simulink subsystem "Battery_Model"  (R2021b)
settings: Solver=VariableStepAuto  StartTime=0.0  StopTime=10.0  RelTol=1e-3
undefined symbols (not defined in the file): Battery, Np_Module
libraries: fl_lib x580, nesl_utility x386, ee_lib x96, simulink x96
(part 4 of 6)

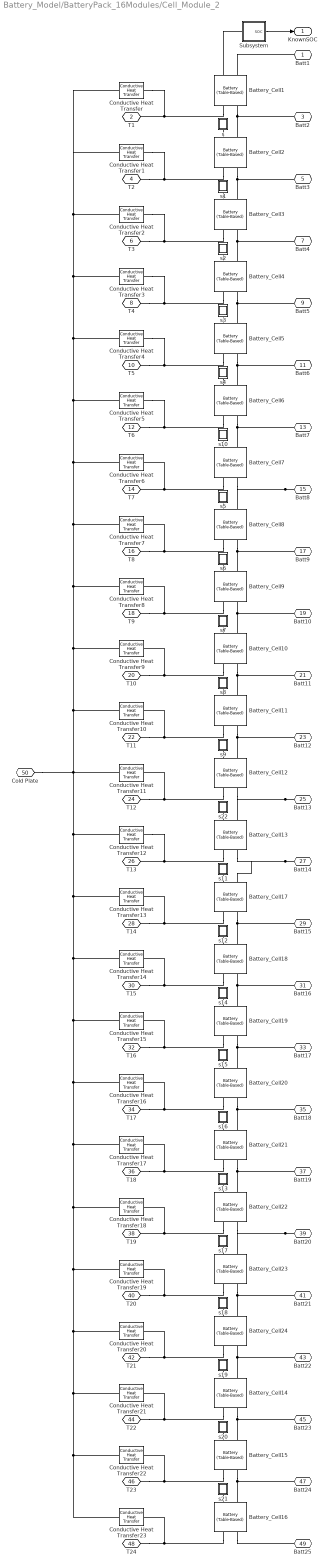
== system Battery_Model/BatteryPack_16Modules/Cell_Module_2 ==
  Battery_Cell{1..24} (24 alike) : ee_lib/Sources/Battery (Table-Based)  Tag={'toolbox/physmod/elec/library/m/ee_lib_parts';'Sources/Battery__Table_Based_/Panasonic/NCR18650BD.xml'}  SOC_vec=Battery.SOC_LUT  T_dependence=ee.enum.temperature_dependence.yes  prm_dir=ee.enum.battery.prm_dir.noCurrentDirectionality  T_vec=Battery.Temperature_LUT degC  V0_mat=Battery.Em_LUT V  V0_vec=[3.01162183959268 3.08575650269622 3.14177499163339 3.18631823552003 3.22334954767724 3.25390136234099 3.27878869705109 3.30070350874259 3.32118523630503 3.33873222862982 3.35681278765286 3.3727103181478 3.38793252475269 3.40246133852855 3.41323877471787 3.42274053961048 3.43230513033606 3.44127066639713 3.45046092538443 3.46050021597496 3.47059444208772 3.47754582201769 3.48403887676592 3.49083263175798 3.49762638675004 3.50414427848956 3.51006189737342 3.51650779121088 3.52300031605604 3.5294928409012 3.53574150484027 3.54126505716735 3.54599126111241 3.55084210438451 3.55569196094666 3.56052372392349 3.56532059653064 3.56979945432131 3.57444121267711 3.57904303346503 3.58364485425295 3.58840361874736 3.5931676308725 3.59914045642067 3.60536834334135 3.61166009904557 3.61797346412467 3.62428682920377 3.63060019428287 3.63762035332317 3.64493091713641 3.65193784155324 3.65894476597006 3.66595169038689 3.67346631195551 3.68205597286888 3.69093403907072 3.69981210527255 3.70876940774879 3.71776352136613 3.72686785650522 3.73538877817079 3.74389655120326 3.7524031927436 3.76046489817023 3.76888762106825 3.7779024493972 3.78684332393235 3.7957841984675 3.80453642296868 3.81235798589345 3.82032795054979 3.82829600796219 3.83626406537459 3.84436267545786 3.8525073311682 3.86057855536852 3.86864977956884 3.87672100376915 3.8849361052788 3.89310639828889 3.90173837211625 3.91095173577988 3.92144530461468 3.93240377767841 3.94373568413835 3.95558619350771 3.96743304428185 3.9792002957498 3.99089798499065 4.00334195302942 4.01527114968024 4.0272843604214 4.03909414300309 4.04916289177822 4.05870791988182 4.06775178122738 4.07651000374835 4.08674414955216 4.1040722856973] V  R0_mat=Battery.R0_LUT/Np_Module Ohm  R0_vec=[0.108383589577359 0.104276452250663 0.0975073630060557 0.0937501268832217 0.0893819468578965 0.085464471367626 0.08175755280038 0.0789657156023766 0.0763700410896049 0.0743500050394976 0.0728433546029721 0.0716898267238282 0.0709947524858037 0.0701675330798173 0.0687296636498531 0.0673712307537144 0.066215812656778 0.0650205672726791 0.0638581443118 0.0632667622677965 0.0628323749302964 0.0619127995096651 0.0610362875653991 0.0603620203223802 0.0596877530793609 0.0589554578065767 0.0582121279560432 0.0577538001128373 0.0573051863053595 0.0568565724978818 0.0563566623767877 0.055788965071129 0.0551527157042777 0.0546601636283963 0.0541676729953156 0.0536763090566326 0.0531776059040765 0.0526119236645948 0.0520712300263528 0.0515036752143958 0.0509361204024388 0.0503587926465561 0.0497811381187243 0.0494179007317461 0.0491061102549 0.0488178197046287 0.0485440631684004 0.0482703066321726 0.0479965500959447 0.0478381475470897 0.0477067926990284 0.0473712163371034 0.0470356399751788 0.0467000636132555 0.0464310667647791 0.0463210072143654 0.0462716139198203 0.0462222206252756 0.0462261199933538 0.0462489440940042 0.0463125045945074 0.0462585966454419 0.046201922872132 0.046144488080849 0.0458836890808221 0.0457208666912199 0.0456935258730669 0.0456707901856075 0.0456480544981481 0.0455856361429716 0.0453236882021848 0.0450859495122442 0.0448483295871047 0.0446107096619652 0.0444608967355156 0.0443618965142365 0.0442474499230245 0.0441330033318126 0.0440185567406002 0.0437935866730954 0.0434800673484186 0.0432636629093239 0.0431695542324042 0.0433145404237085 0.043616651255713 0.0439115402259742 0.0443155176840522 0.0447170344474341 0.0451426585495343 0.0455784262459233 0.0461653340876942 0.0463666936277911 0.0465478472510501 0.0466774333752156 0.0460938543815081 0.045231226285297 0.0442160431848739 0.0431407757562075 0.0415552249991693 0.0395514196760085] Ohm  R0_dis_mat=[0.03 0.015 0.002;0.04 0.017 0.008;0.039 0.012 0.006;0.027 0.013 0.021] % Parameter not set Ohm  R0_dis_vec=[0.015 0.017 0.012 0.013] % Parameter not set Ohm  R0_ch_mat=[0.03 0.015 0.002;0.04 0.017 0.008;0.039 0.012 0.006;0.027 0.013 0.021] % Parameter not set Ohm  R0_ch_vec=[0.015 0.017 0.012 0.013] % Parameter not set Ohm  AH_vec=Battery.Capacity_LUT*Np_Module hr*A  AH=3.03732766876938 hr*A  prm_leak=ee.enum.battery.prm_leak.disabled  Rleak_vec=[8000 7000 6000] % Parameter not set Ohm  Rleak=7000 % Parameter not set Ohm  extrapolation_option=ee.enum.extrapolation.nearest  prm_dyn=ee.enum.battery.prm_dyn.rc1  R1_mat=Battery.R1_LUT/Np_Module Ohm  R1_vec=[0.076 0.022 0.007 0.043] % Parameter not set Ohm  tau1_mat=(Battery.R1_LUT/Np_Module).*(Battery.C1_LUT*Np_Module) s  tau1_vec=[148 110 27 22] % Parameter not set s  R2_mat=[0.014 0.382 0.407;0.028 0.006 0.007;0.014 0.007 0.006;0.333 0.956 0.912] % Parameter not set Ohm  R2_vec=[0.382 0.006 0.007 0.956] % Parameter not set Ohm  tau2_mat=[1 44 5644;11 24 506;2 14 330;3310 13419 30216] % Parameter not set s  tau2_vec=[44 24 14 13419] % Parameter not set s  R3_mat=[0.014 0.382 0.407;0.028 0.006 0.007;0.014 0.007 0.006;0.333 0.956 0.912] % Parameter not set Ohm  R3_vec=[0.382 0.006 0.007 0.956] % Parameter not set Ohm  tau3_mat=[1 44 5644;11 24 506;2 14 330;3310 13419 30216] % Parameter not set s  tau3_vec=[44 24 14 13419] % Parameter not set s  R4_mat=[0.014 0.382 0.407;0.028 0.006 0.007;0.014 0.007 0.006;0.333 0.956 0.912] % Parameter not set Ohm  R4_vec=[0.382 0.006 0.007 0.956] % Parameter not set Ohm  tau4_mat=[1 44 5644;11 24 506;2 14 330;3310 13419 30216] % Parameter not set s  tau4_vec=[44 24 14 13419] % Parameter not set s  R5_mat=[0.014 0.382 0.407;0.028 0.006 0.007;0.014 0.007 0.006;0.333 0.956 0.912] % Parameter not set Ohm  R5_vec=[0.382 0.006 0.007 0.956] % Parameter not set Ohm  tau5_mat=[1 44 5644;11 24 506;2 14 330;3310 13419 30216] % Parameter not set s  tau5_vec=[44 24 14 13419] % Parameter not set s  prm_fade=ee.enum.battery.prm_fade.tableN  N0=100 % Parameter not set  dV0=0 % Parameter not set  dR0=0 % Parameter not set  dAH=0 % Parameter not set  dRleak=0 % Parameter not set  dR1=0 % Parameter not set  dR2=0 % Parameter not set  dR3=0 % Parameter not set  dR4=0 % Parameter not set  dR5=0 % Parameter not set  N0vec=Battery.DischargeCycle_LUT  Tfadevec=[298.15 323.15] % Parameter not set K  dV0vec=Battery.deltaEm_LUT  dR0vec=[0;0;0;0;0;0;0;0;0;0;0;0;0;0;0;0;0;0;0;0;0;0;0;0;0;0;0;0;0;0;0;0;0;0;0;0;0;0;0;0;0;0;0;0;0;0;0;0;0;0;0;0;0;0;0;0;0;0;0;0;0;0;0;0;0;0;0;0;0;0;0;0;0;0;0;0;0;0;0;0] % Parameter not set  dAHvec=Battery.deltaCapacity_LUT  dRleakvec=[0 0 0] % Parameter not set  dR1vec=[0;0;0;0;0;0;0;0;0;0;0;0;0;0;0;0;0;0;0;0;0;0;0;0;0;0;0;0;0;0;0;0;0;0;0;0;0;0;0;0;0;0;0;0;0;0;0;0;0;0;0;0;0;0;0;0;0;0;0;0;0;0;0;0;0;0;0;0;0;0;0;0;0;0;0;0;0;0;0;0] % Parameter not set  dR2vec=[0 0 0] % Parameter not set  dR3vec=[0 0 0] % Parameter not set  dR4vec=[0 0 0] % Parameter not set  dR5vec=[0 0 0] % Parameter not set  dV0mat=[0 0;0 0;0 0] % Parameter not set  dR0mat=[0 0;0 0;0 0] % Parameter not set  dAHmat=[0 0;0 0;0 0] % Parameter not set  dRleakmat=[0 0;0 0;0 0] % Parameter not set  dR1mat=[0 0;0 0;0 0] % Parameter not set  dR2mat=[0 0;0 0;0 0] % Parameter not set  dR3mat=[0 0;0 0;0 0] % Parameter not set  dR4mat=[0 0;0 0;0 0] % Parameter not set  dR5mat=[0 0;0 0;0 0] % Parameter not set  prm_age=ee.enum.battery.prm_age.disabled  prm_age_OCV=ee.enum.battery.prm_age_OCV.OCV  OCV_age=0.9  SOC_age=0.6  storage_dt_age_vec=[0] d  storage_T_age_vec=[273] K  OCV_scaling_age=2.2134e6  OCV_offset_age=1.632e6  temp_exp_age=0.515833569 V  t_exp_age=0.75  T_age_vec=[273.15, 298.15, 323.15] K  dt_age_vec=[90, 180, 270, 360] d  dR0_age_vec=[0, 0, 0]  t_meas_dR0_age=100 d  dR0_age_mat=[0, 0, 0; 0, 0, 0; 0, 0, 0; 0, 0, 0]  temperature=BattTempInit degC  i_specify=off  i_priority=None  i=0 A  i_nominal_specify=off  i_nominal_unit=A  i_nominal_value=1  v_specify=off  v_priority=None  v=0 V  v_nominal_specify=off  v_nominal_unit=V  v_nominal_value=1  stateOfCharge_specify=on  stateOfCharge_priority=High  stateOfCharge=BattSocInit  stateOfCharge_nominal_specify=off  stateOfCharge_nominal_unit=1  stateOfCharge_nominal_value=1  num_cycles_specify=off  num_cycles_priority=High  num_cycles=0  num_cycles_nominal_specify=off  num_cycles_nominal_unit=1  num_cycles_nominal_value=1  thermal_mass=Battery.ThermalMass*Np_Module J/K  temperature_specify=on  temperature_priority=High  temperature_nominal_specify=off  temperature_nominal_unit=K  temperature_nominal_value=1
      settings: AttributesFormatString=Panasonic:NCR18650BD  SourceProductBaseCode=PS  InternalSimscapePortConfiguration="{\"Bottom\":[],\"Left\":[{\"id\":\"p\",\"label\":\"+\",\"type\":\"foundation.electrical.electrical\"},{\"id\":\"soc\",\"label\":\"SOC\",\"type\":\"output\"}],\"Right\":[{\"id\":\"n\",\"label\":\"-\",\"type\":\"foundation.electrical.electrical\"},{\"id\":\"H\",\"label\":\"H\",\"type\":\"foundation.thermal.thermal\"}],\"Top\":[]}"
  Conductive Heat Transfer{,1..23} (24 alike) : fl_lib/Thermal/Thermal Elements/Conductive Heat Transfer  area=Battery.cell_area*Np_Module m^2  thickness=Battery.cond_thickness m  th_cond=Battery.thermal_conductivity W/(m*K)  T_specify=off  T_priority=None  T=0 K  T_nominal_specify=off  T_nominal_unit=K  T_nominal_value=1  Q_specify=off  Q_priority=None  Q=0 W  Q_nominal_specify=off  Q_nominal_unit=W  Q_nominal_value=1
  Subsystem : Subsystem
  s : Subsystem
  s1 : Subsystem
  s10 : Subsystem
  s11 : Subsystem
  s12 : Subsystem
  s13 : Subsystem
  s14 : Subsystem
  s15 : Subsystem
  s16 : Subsystem
  s17 : Subsystem
  s18 : Subsystem
  s19 : Subsystem
  s2 : Subsystem
  s20 : Subsystem
  s21 : Subsystem
  s22 : Subsystem
  s3 : Subsystem
  s4 : Subsystem
  s5 : Subsystem
  s6 : Subsystem
  s7 : Subsystem
  s8 : Subsystem
  s9 : Subsystem
  Batt1 : PMIOPort  Side=Right
  T1 : PMIOPort  Port=2  Side=Right
  Batt2 : PMIOPort  Port=3  Side=Right
  T2 : PMIOPort  Port=4  Side=Right
  Batt3 : PMIOPort  Port=5  Side=Right
  T3 : PMIOPort  Port=6  Side=Right
  Batt4 : PMIOPort  Port=7  Side=Right
  T4 : PMIOPort  Port=8  Side=Right
  Batt5 : PMIOPort  Port=9  Side=Right
  T5 : PMIOPort  Port=10  Side=Right
  Batt6 : PMIOPort  Port=11  Side=Right
  T6 : PMIOPort  Port=12  Side=Right
  Batt7 : PMIOPort  Port=13  Side=Right
  T7 : PMIOPort  Port=14  Side=Right
  Batt8 : PMIOPort  Port=15  Side=Right
  T8 : PMIOPort  Port=16  Side=Right
  Batt9 : PMIOPort  Port=17  Side=Right
  T9 : PMIOPort  Port=18  Side=Right
  Batt10 : PMIOPort  Port=19  Side=Right
  T10 : PMIOPort  Port=20  Side=Right
  Batt11 : PMIOPort  Port=21  Side=Right
  T11 : PMIOPort  Port=22  Side=Right
  Batt12 : PMIOPort  Port=23  Side=Right
  T12 : PMIOPort  Port=24  Side=Right
  Batt13 : PMIOPort  Port=25  Side=Right
  T13 : PMIOPort  Port=26  Side=Right
  Batt14 : PMIOPort  Port=27  Side=Right
  T14 : PMIOPort  Port=28  Side=Right
  Batt15 : PMIOPort  Port=29  Side=Right
  T15 : PMIOPort  Port=30  Side=Right
  Batt16 : PMIOPort  Port=31  Side=Right
  T16 : PMIOPort  Port=32  Side=Right
  Batt17 : PMIOPort  Port=33  Side=Right
  T17 : PMIOPort  Port=34  Side=Right
  Batt18 : PMIOPort  Port=35  Side=Right
  T18 : PMIOPort  Port=36  Side=Right
  Batt19 : PMIOPort  Port=37  Side=Right
  T19 : PMIOPort  Port=38  Side=Right
  Batt20 : PMIOPort  Port=39  Side=Right
  T20 : PMIOPort  Port=40  Side=Right
  Batt21 : PMIOPort  Port=41  Side=Right
  T21 : PMIOPort  Port=42  Side=Right
  Batt22 : PMIOPort  Port=43  Side=Right
  T22 : PMIOPort  Port=44  Side=Right
  Batt23 : PMIOPort  Port=45  Side=Right
  T23 : PMIOPort  Port=46  Side=Right
  Batt24 : PMIOPort  Port=47  Side=Right
  T24 : PMIOPort  Port=48  Side=Right
  Batt25 : PMIOPort  Port=49  Side=Right
  Cold Plate : PMIOPort  Port=50  Side=Left
  KnownSOC : Outport
  wires:
  Subsystem/1(soc) -> KnownSOC/1
  connections:
  Battery_Cell13/LConn2 -- s22/LConn1
  Battery_Cell24/LConn2 -- s18/LConn1
  Battery_Cell16/RConn1 -- Batt25/RConn1
  Battery_Cell18/LConn2 -- s12/LConn1
  Battery_Cell22/LConn2 -- s13/LConn1
  Battery_Cell17/LConn2 -- s11/LConn1
  Battery_Cell15/LConn2 -- s20/LConn1
  Battery_Cell21/LConn2 -- s16/LConn1
  Battery_Cell23/LConn2 -- s17/LConn1
  Battery_Cell16/LConn2 -- s21/LConn1
  Battery_Cell19/LConn2 -- s14/LConn1
  Battery_Cell20/LConn2 -- s15/LConn1
  Battery_Cell14/LConn2 -- s19/LConn1
  Battery_Cell17/RConn1 -- Batt15/RConn1 -- Battery_Cell18/LConn1
  Battery_Cell15/RConn2 -- Conductive Heat Transfer22/LConn1 -- T23/RConn1
  Battery_Cell22/RConn2 -- Conductive Heat Transfer18/LConn1 -- T19/RConn1
  Battery_Cell21/RConn1 -- Batt19/RConn1 -- Battery_Cell22/LConn1
  Battery_Cell14/LConn1 -- Batt22/RConn1 -- Battery_Cell24/RConn1
  Battery_Cell20/RConn2 -- Conductive Heat Transfer16/LConn1 -- T17/RConn1
  Battery_Cell13/RConn2 -- Conductive Heat Transfer12/LConn1 -- T13/RConn1
  Battery_Cell18/RConn2 -- Conductive Heat Transfer14/LConn1 -- T15/RConn1
  Battery_Cell16/RConn2 -- Conductive Heat Transfer23/LConn1 -- T24/RConn1
  Battery_Cell14/RConn2 -- Conductive Heat Transfer21/LConn1 -- T22/RConn1
  Battery_Cell20/RConn1 -- Batt18/RConn1 -- Battery_Cell21/LConn1
  Battery_Cell14/RConn1 -- Batt23/RConn1 -- Battery_Cell15/LConn1
  Battery_Cell19/RConn1 -- Batt17/RConn1 -- Battery_Cell20/LConn1
  Battery_Cell23/RConn2 -- Conductive Heat Transfer19/LConn1 -- T20/RConn1
  Battery_Cell24/RConn2 -- Conductive Heat Transfer20/LConn1 -- T21/RConn1
  Battery_Cell17/RConn2 -- Conductive Heat Transfer13/LConn1 -- T14/RConn1
  Battery_Cell15/RConn1 -- Batt24/RConn1 -- Battery_Cell16/LConn1
  Battery_Cell19/LConn1 -- Batt16/RConn1 -- Battery_Cell18/RConn1
  Battery_Cell19/RConn2 -- Conductive Heat Transfer15/LConn1 -- T16/RConn1
  Battery_Cell23/RConn1 -- Batt21/RConn1 -- Battery_Cell24/LConn1
  Battery_Cell21/RConn2 -- Conductive Heat Transfer17/LConn1 -- T18/RConn1
  Batt14/RConn1 -- Battery_Cell17/LConn1 -- Battery_Cell13/RConn1
  Batt20/RConn1 -- Battery_Cell23/LConn1 -- Battery_Cell22/RConn1
  Battery_Cell7/LConn2 -- s10/LConn1
  Battery_Cell9/LConn2 -- s6/LConn1
  Battery_Cell8/LConn2 -- s5/LConn1
  Battery_Cell12/LConn2 -- s9/LConn1
  Battery_Cell10/LConn2 -- s7/LConn1
  Batt13/RConn1 -- Battery_Cell13/LConn1 -- Battery_Cell12/RConn1
  Battery_Cell11/LConn2 -- s8/LConn1
  Battery_Cell9/RConn2 -- Conductive Heat Transfer8/LConn1 -- T9/RConn1
  Battery_Cell8/RConn2 -- Conductive Heat Transfer7/LConn1 -- T8/RConn1
  Battery_Cell11/RConn2 -- Conductive Heat Transfer10/LConn1 -- T11/RConn1
  Battery_Cell10/LConn1 -- Batt10/RConn1 -- Battery_Cell9/RConn1
  Battery_Cell10/RConn1 -- Batt11/RConn1 -- Battery_Cell11/LConn1
  Battery_Cell10/RConn2 -- Conductive Heat Transfer9/LConn1 -- T10/RConn1
  Battery_Cell8/RConn1 -- Batt9/RConn1 -- Battery_Cell9/LConn1
  Battery_Cell11/RConn1 -- Batt12/RConn1 -- Battery_Cell12/LConn1
  Battery_Cell12/RConn2 -- Conductive Heat Transfer11/LConn1 -- T12/RConn1
  Batt8/RConn1 -- Battery_Cell7/RConn1 -- Battery_Cell8/LConn1
  Battery_Cell7/RConn2 -- Conductive Heat Transfer6/LConn1 -- T7/RConn1
  Batt5/RConn1 -- Battery_Cell5/LConn1 -- Battery_Cell4/RConn1
  Batt6/RConn1 -- Battery_Cell6/LConn1 -- Battery_Cell5/RConn1
  Batt4/RConn1 -- Battery_Cell3/RConn1 -- Battery_Cell4/LConn1
  Battery_Cell1/RConn2 -- Conductive Heat Transfer/LConn1 -- T1/RConn1
  Battery_Cell5/RConn2 -- Conductive Heat Transfer4/LConn1 -- T5/RConn1
  Battery_Cell1/RConn1 -- Battery_Cell2/LConn1 -- Batt2/RConn1
  Battery_Cell6/RConn2 -- Conductive Heat Transfer5/LConn1 -- T6/RConn1
  Conductive Heat Transfer22/RConn1 -- Conductive Heat Transfer23/RConn1 -- Conductive Heat Transfer21/RConn1 -- Conductive Heat Transfer20/RConn1 -- Conductive Heat Transfer19/RConn1 -- Conductive Heat Transfer18/RConn1 -- Conductive Heat Transfer17/RConn1 -- Conductive Heat Transfer16/RConn1 -- Conductive Heat Transfer15/RConn1 -- Conductive Heat Transfer14/RConn1 -- Conductive Heat Transfer13/RConn1 -- Conductive Heat Transfer11/RConn1 -- Cold Plate/RConn1 -- Conductive Heat Transfer10/RConn1 -- Conductive Heat Transfer9/RConn1 -- Conductive Heat Transfer8/RConn1 -- Conductive Heat Transfer7/RConn1 -- Conductive Heat Transfer6/RConn1 -- Conductive Heat Transfer5/RConn1 -- Conductive Heat Transfer4/RConn1 -- Conductive Heat Transfer/RConn1 -- Conductive Heat Transfer1/RConn1 -- Conductive Heat Transfer2/RConn1 -- Conductive Heat Transfer3/RConn1 -- Conductive Heat Transfer12/RConn1
  Battery_Cell7/LConn1 -- Batt7/RConn1 -- Battery_Cell6/RConn1
  Batt1/RConn1 -- Battery_Cell1/LConn1
  Batt3/RConn1 -- Battery_Cell3/LConn1 -- Battery_Cell2/RConn1
  Battery_Cell1/LConn2 -- Subsystem/LConn1
  Battery_Cell2/LConn2 -- s/LConn1
  Battery_Cell3/LConn2 -- s1/LConn1
  Battery_Cell4/LConn2 -- s2/LConn1
  Battery_Cell5/LConn2 -- s3/LConn1
  Battery_Cell6/LConn2 -- s4/LConn1
  Battery_Cell3/RConn2 -- Conductive Heat Transfer2/LConn1 -- T3/RConn1
  Battery_Cell2/RConn2 -- Conductive Heat Transfer1/LConn1 -- T2/RConn1
  Battery_Cell4/RConn2 -- Conductive Heat Transfer3/LConn1 -- T4/RConn1

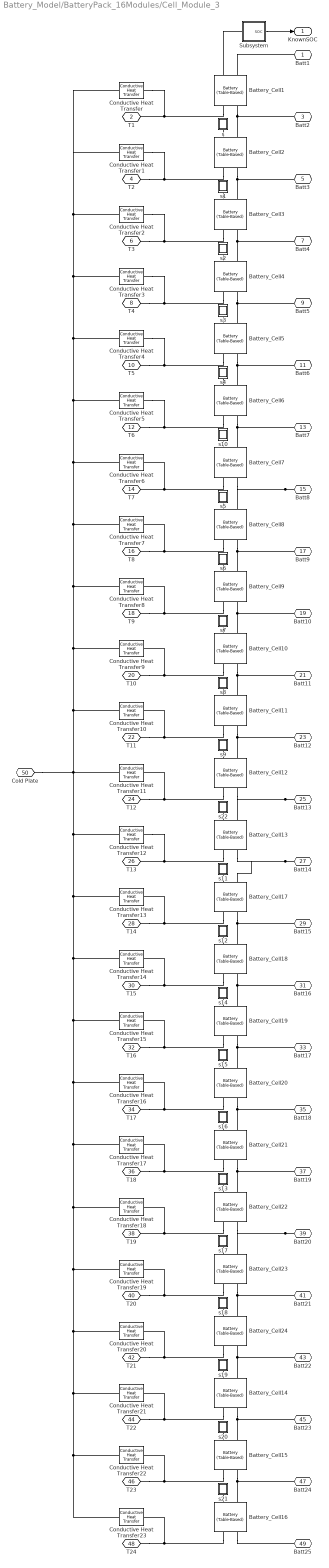
== system Battery_Model/BatteryPack_16Modules/Cell_Module_3 ==
  Battery_Cell{1..24} (24 alike) : ee_lib/Sources/Battery (Table-Based)  Tag={'toolbox/physmod/elec/library/m/ee_lib_parts';'Sources/Battery__Table_Based_/Panasonic/NCR18650BD.xml'}  SOC_vec=Battery.SOC_LUT  T_dependence=ee.enum.temperature_dependence.yes  prm_dir=ee.enum.battery.prm_dir.noCurrentDirectionality  T_vec=Battery.Temperature_LUT degC  V0_mat=Battery.Em_LUT V  V0_vec=[3.01162183959268 3.08575650269622 3.14177499163339 3.18631823552003 3.22334954767724 3.25390136234099 3.27878869705109 3.30070350874259 3.32118523630503 3.33873222862982 3.35681278765286 3.3727103181478 3.38793252475269 3.40246133852855 3.41323877471787 3.42274053961048 3.43230513033606 3.44127066639713 3.45046092538443 3.46050021597496 3.47059444208772 3.47754582201769 3.48403887676592 3.49083263175798 3.49762638675004 3.50414427848956 3.51006189737342 3.51650779121088 3.52300031605604 3.5294928409012 3.53574150484027 3.54126505716735 3.54599126111241 3.55084210438451 3.55569196094666 3.56052372392349 3.56532059653064 3.56979945432131 3.57444121267711 3.57904303346503 3.58364485425295 3.58840361874736 3.5931676308725 3.59914045642067 3.60536834334135 3.61166009904557 3.61797346412467 3.62428682920377 3.63060019428287 3.63762035332317 3.64493091713641 3.65193784155324 3.65894476597006 3.66595169038689 3.67346631195551 3.68205597286888 3.69093403907072 3.69981210527255 3.70876940774879 3.71776352136613 3.72686785650522 3.73538877817079 3.74389655120326 3.7524031927436 3.76046489817023 3.76888762106825 3.7779024493972 3.78684332393235 3.7957841984675 3.80453642296868 3.81235798589345 3.82032795054979 3.82829600796219 3.83626406537459 3.84436267545786 3.8525073311682 3.86057855536852 3.86864977956884 3.87672100376915 3.8849361052788 3.89310639828889 3.90173837211625 3.91095173577988 3.92144530461468 3.93240377767841 3.94373568413835 3.95558619350771 3.96743304428185 3.9792002957498 3.99089798499065 4.00334195302942 4.01527114968024 4.0272843604214 4.03909414300309 4.04916289177822 4.05870791988182 4.06775178122738 4.07651000374835 4.08674414955216 4.1040722856973] V  R0_mat=Battery.R0_LUT/Np_Module Ohm  R0_vec=[0.108383589577359 0.104276452250663 0.0975073630060557 0.0937501268832217 0.0893819468578965 0.085464471367626 0.08175755280038 0.0789657156023766 0.0763700410896049 0.0743500050394976 0.0728433546029721 0.0716898267238282 0.0709947524858037 0.0701675330798173 0.0687296636498531 0.0673712307537144 0.066215812656778 0.0650205672726791 0.0638581443118 0.0632667622677965 0.0628323749302964 0.0619127995096651 0.0610362875653991 0.0603620203223802 0.0596877530793609 0.0589554578065767 0.0582121279560432 0.0577538001128373 0.0573051863053595 0.0568565724978818 0.0563566623767877 0.055788965071129 0.0551527157042777 0.0546601636283963 0.0541676729953156 0.0536763090566326 0.0531776059040765 0.0526119236645948 0.0520712300263528 0.0515036752143958 0.0509361204024388 0.0503587926465561 0.0497811381187243 0.0494179007317461 0.0491061102549 0.0488178197046287 0.0485440631684004 0.0482703066321726 0.0479965500959447 0.0478381475470897 0.0477067926990284 0.0473712163371034 0.0470356399751788 0.0467000636132555 0.0464310667647791 0.0463210072143654 0.0462716139198203 0.0462222206252756 0.0462261199933538 0.0462489440940042 0.0463125045945074 0.0462585966454419 0.046201922872132 0.046144488080849 0.0458836890808221 0.0457208666912199 0.0456935258730669 0.0456707901856075 0.0456480544981481 0.0455856361429716 0.0453236882021848 0.0450859495122442 0.0448483295871047 0.0446107096619652 0.0444608967355156 0.0443618965142365 0.0442474499230245 0.0441330033318126 0.0440185567406002 0.0437935866730954 0.0434800673484186 0.0432636629093239 0.0431695542324042 0.0433145404237085 0.043616651255713 0.0439115402259742 0.0443155176840522 0.0447170344474341 0.0451426585495343 0.0455784262459233 0.0461653340876942 0.0463666936277911 0.0465478472510501 0.0466774333752156 0.0460938543815081 0.045231226285297 0.0442160431848739 0.0431407757562075 0.0415552249991693 0.0395514196760085] Ohm  R0_dis_mat=[0.03 0.015 0.002;0.04 0.017 0.008;0.039 0.012 0.006;0.027 0.013 0.021] % Parameter not set Ohm  R0_dis_vec=[0.015 0.017 0.012 0.013] % Parameter not set Ohm  R0_ch_mat=[0.03 0.015 0.002;0.04 0.017 0.008;0.039 0.012 0.006;0.027 0.013 0.021] % Parameter not set Ohm  R0_ch_vec=[0.015 0.017 0.012 0.013] % Parameter not set Ohm  AH_vec=Battery.Capacity_LUT*Np_Module hr*A  AH=3.03732766876938 hr*A  prm_leak=ee.enum.battery.prm_leak.disabled  Rleak_vec=[8000 7000 6000] % Parameter not set Ohm  Rleak=7000 % Parameter not set Ohm  extrapolation_option=ee.enum.extrapolation.nearest  prm_dyn=ee.enum.battery.prm_dyn.rc1  R1_mat=Battery.R1_LUT/Np_Module Ohm  R1_vec=[0.076 0.022 0.007 0.043] % Parameter not set Ohm  tau1_mat=(Battery.R1_LUT/Np_Module).*(Battery.C1_LUT*Np_Module) s  tau1_vec=[148 110 27 22] % Parameter not set s  R2_mat=[0.014 0.382 0.407;0.028 0.006 0.007;0.014 0.007 0.006;0.333 0.956 0.912] % Parameter not set Ohm  R2_vec=[0.382 0.006 0.007 0.956] % Parameter not set Ohm  tau2_mat=[1 44 5644;11 24 506;2 14 330;3310 13419 30216] % Parameter not set s  tau2_vec=[44 24 14 13419] % Parameter not set s  R3_mat=[0.014 0.382 0.407;0.028 0.006 0.007;0.014 0.007 0.006;0.333 0.956 0.912] % Parameter not set Ohm  R3_vec=[0.382 0.006 0.007 0.956] % Parameter not set Ohm  tau3_mat=[1 44 5644;11 24 506;2 14 330;3310 13419 30216] % Parameter not set s  tau3_vec=[44 24 14 13419] % Parameter not set s  R4_mat=[0.014 0.382 0.407;0.028 0.006 0.007;0.014 0.007 0.006;0.333 0.956 0.912] % Parameter not set Ohm  R4_vec=[0.382 0.006 0.007 0.956] % Parameter not set Ohm  tau4_mat=[1 44 5644;11 24 506;2 14 330;3310 13419 30216] % Parameter not set s  tau4_vec=[44 24 14 13419] % Parameter not set s  R5_mat=[0.014 0.382 0.407;0.028 0.006 0.007;0.014 0.007 0.006;0.333 0.956 0.912] % Parameter not set Ohm  R5_vec=[0.382 0.006 0.007 0.956] % Parameter not set Ohm  tau5_mat=[1 44 5644;11 24 506;2 14 330;3310 13419 30216] % Parameter not set s  tau5_vec=[44 24 14 13419] % Parameter not set s  prm_fade=ee.enum.battery.prm_fade.tableN  N0=100 % Parameter not set  dV0=0 % Parameter not set  dR0=0 % Parameter not set  dAH=0 % Parameter not set  dRleak=0 % Parameter not set  dR1=0 % Parameter not set  dR2=0 % Parameter not set  dR3=0 % Parameter not set  dR4=0 % Parameter not set  dR5=0 % Parameter not set  N0vec=Battery.DischargeCycle_LUT  Tfadevec=[298.15 323.15] % Parameter not set K  dV0vec=Battery.deltaEm_LUT  dR0vec=[0;0;0;0;0;0;0;0;0;0;0;0;0;0;0;0;0;0;0;0;0;0;0;0;0;0;0;0;0;0;0;0;0;0;0;0;0;0;0;0;0;0;0;0;0;0;0;0;0;0;0;0;0;0;0;0;0;0;0;0;0;0;0;0;0;0;0;0;0;0;0;0;0;0;0;0;0;0;0;0] % Parameter not set  dAHvec=Battery.deltaCapacity_LUT  dRleakvec=[0 0 0] % Parameter not set  dR1vec=[0;0;0;0;0;0;0;0;0;0;0;0;0;0;0;0;0;0;0;0;0;0;0;0;0;0;0;0;0;0;0;0;0;0;0;0;0;0;0;0;0;0;0;0;0;0;0;0;0;0;0;0;0;0;0;0;0;0;0;0;0;0;0;0;0;0;0;0;0;0;0;0;0;0;0;0;0;0;0;0] % Parameter not set  dR2vec=[0 0 0] % Parameter not set  dR3vec=[0 0 0] % Parameter not set  dR4vec=[0 0 0] % Parameter not set  dR5vec=[0 0 0] % Parameter not set  dV0mat=[0 0;0 0;0 0] % Parameter not set  dR0mat=[0 0;0 0;0 0] % Parameter not set  dAHmat=[0 0;0 0;0 0] % Parameter not set  dRleakmat=[0 0;0 0;0 0] % Parameter not set  dR1mat=[0 0;0 0;0 0] % Parameter not set  dR2mat=[0 0;0 0;0 0] % Parameter not set  dR3mat=[0 0;0 0;0 0] % Parameter not set  dR4mat=[0 0;0 0;0 0] % Parameter not set  dR5mat=[0 0;0 0;0 0] % Parameter not set  prm_age=ee.enum.battery.prm_age.disabled  prm_age_OCV=ee.enum.battery.prm_age_OCV.OCV  OCV_age=0.9  SOC_age=0.6  storage_dt_age_vec=[0] d  storage_T_age_vec=[273] K  OCV_scaling_age=2.2134e6  OCV_offset_age=1.632e6  temp_exp_age=0.515833569 V  t_exp_age=0.75  T_age_vec=[273.15, 298.15, 323.15] K  dt_age_vec=[90, 180, 270, 360] d  dR0_age_vec=[0, 0, 0]  t_meas_dR0_age=100 d  dR0_age_mat=[0, 0, 0; 0, 0, 0; 0, 0, 0; 0, 0, 0]  temperature=BattTempInit degC  i_specify=off  i_priority=None  i=0 A  i_nominal_specify=off  i_nominal_unit=A  i_nominal_value=1  v_specify=off  v_priority=None  v=0 V  v_nominal_specify=off  v_nominal_unit=V  v_nominal_value=1  stateOfCharge_specify=on  stateOfCharge_priority=High  stateOfCharge=BattSocInit  stateOfCharge_nominal_specify=off  stateOfCharge_nominal_unit=1  stateOfCharge_nominal_value=1  num_cycles_specify=off  num_cycles_priority=High  num_cycles=0  num_cycles_nominal_specify=off  num_cycles_nominal_unit=1  num_cycles_nominal_value=1  thermal_mass=Battery.ThermalMass*Np_Module J/K  temperature_specify=on  temperature_priority=High  temperature_nominal_specify=off  temperature_nominal_unit=K  temperature_nominal_value=1
      settings: AttributesFormatString=Panasonic:NCR18650BD  SourceProductBaseCode=PS  InternalSimscapePortConfiguration="{\"Bottom\":[],\"Left\":[{\"id\":\"p\",\"label\":\"+\",\"type\":\"foundation.electrical.electrical\"},{\"id\":\"soc\",\"label\":\"SOC\",\"type\":\"output\"}],\"Right\":[{\"id\":\"n\",\"label\":\"-\",\"type\":\"foundation.electrical.electrical\"},{\"id\":\"H\",\"label\":\"H\",\"type\":\"foundation.thermal.thermal\"}],\"Top\":[]}"
  Conductive Heat Transfer{,1..23} (24 alike) : fl_lib/Thermal/Thermal Elements/Conductive Heat Transfer  area=Battery.cell_area*Np_Module m^2  thickness=Battery.cond_thickness m  th_cond=Battery.thermal_conductivity W/(m*K)  T_specify=off  T_priority=None  T=0 K  T_nominal_specify=off  T_nominal_unit=K  T_nominal_value=1  Q_specify=off  Q_priority=None  Q=0 W  Q_nominal_specify=off  Q_nominal_unit=W  Q_nominal_value=1
  Subsystem : Subsystem
  s : Subsystem
  s1 : Subsystem
  s10 : Subsystem
  s11 : Subsystem
  s12 : Subsystem
  s13 : Subsystem
  s14 : Subsystem
  s15 : Subsystem
  s16 : Subsystem
  s17 : Subsystem
  s18 : Subsystem
  s19 : Subsystem
  s2 : Subsystem
  s20 : Subsystem
  s21 : Subsystem
  s22 : Subsystem
  s3 : Subsystem
  s4 : Subsystem
  s5 : Subsystem
  s6 : Subsystem
  s7 : Subsystem
  s8 : Subsystem
  s9 : Subsystem
  Batt1 : PMIOPort  Side=Right
  T1 : PMIOPort  Port=2  Side=Right
  Batt2 : PMIOPort  Port=3  Side=Right
  T2 : PMIOPort  Port=4  Side=Right
  Batt3 : PMIOPort  Port=5  Side=Right
  T3 : PMIOPort  Port=6  Side=Right
  Batt4 : PMIOPort  Port=7  Side=Right
  T4 : PMIOPort  Port=8  Side=Right
  Batt5 : PMIOPort  Port=9  Side=Right
  T5 : PMIOPort  Port=10  Side=Right
  Batt6 : PMIOPort  Port=11  Side=Right
  T6 : PMIOPort  Port=12  Side=Right
  Batt7 : PMIOPort  Port=13  Side=Right
  T7 : PMIOPort  Port=14  Side=Right
  Batt8 : PMIOPort  Port=15  Side=Right
  T8 : PMIOPort  Port=16  Side=Right
  Batt9 : PMIOPort  Port=17  Side=Right
  T9 : PMIOPort  Port=18  Side=Right
  Batt10 : PMIOPort  Port=19  Side=Right
  T10 : PMIOPort  Port=20  Side=Right
  Batt11 : PMIOPort  Port=21  Side=Right
  T11 : PMIOPort  Port=22  Side=Right
  Batt12 : PMIOPort  Port=23  Side=Right
  T12 : PMIOPort  Port=24  Side=Right
  Batt13 : PMIOPort  Port=25  Side=Right
  T13 : PMIOPort  Port=26  Side=Right
  Batt14 : PMIOPort  Port=27  Side=Right
  T14 : PMIOPort  Port=28  Side=Right
  Batt15 : PMIOPort  Port=29  Side=Right
  T15 : PMIOPort  Port=30  Side=Right
  Batt16 : PMIOPort  Port=31  Side=Right
  T16 : PMIOPort  Port=32  Side=Right
  Batt17 : PMIOPort  Port=33  Side=Right
  T17 : PMIOPort  Port=34  Side=Right
  Batt18 : PMIOPort  Port=35  Side=Right
  T18 : PMIOPort  Port=36  Side=Right
  Batt19 : PMIOPort  Port=37  Side=Right
  T19 : PMIOPort  Port=38  Side=Right
  Batt20 : PMIOPort  Port=39  Side=Right
  T20 : PMIOPort  Port=40  Side=Right
  Batt21 : PMIOPort  Port=41  Side=Right
  T21 : PMIOPort  Port=42  Side=Right
  Batt22 : PMIOPort  Port=43  Side=Right
  T22 : PMIOPort  Port=44  Side=Right
  Batt23 : PMIOPort  Port=45  Side=Right
  T23 : PMIOPort  Port=46  Side=Right
  Batt24 : PMIOPort  Port=47  Side=Right
  T24 : PMIOPort  Port=48  Side=Right
  Batt25 : PMIOPort  Port=49  Side=Right
  Cold Plate : PMIOPort  Port=50  Side=Left
  KnownSOC : Outport
  wires:
  Subsystem/1(soc) -> KnownSOC/1
  connections:
  Battery_Cell13/LConn2 -- s22/LConn1
  Battery_Cell24/LConn2 -- s18/LConn1
  Battery_Cell16/RConn1 -- Batt25/RConn1
  Battery_Cell18/LConn2 -- s12/LConn1
  Battery_Cell22/LConn2 -- s13/LConn1
  Battery_Cell17/LConn2 -- s11/LConn1
  Battery_Cell15/LConn2 -- s20/LConn1
  Battery_Cell21/LConn2 -- s16/LConn1
  Battery_Cell23/LConn2 -- s17/LConn1
  Battery_Cell16/LConn2 -- s21/LConn1
  Battery_Cell19/LConn2 -- s14/LConn1
  Battery_Cell20/LConn2 -- s15/LConn1
  Battery_Cell14/LConn2 -- s19/LConn1
  Battery_Cell17/RConn1 -- Batt15/RConn1 -- Battery_Cell18/LConn1
  Battery_Cell15/RConn2 -- Conductive Heat Transfer22/LConn1 -- T23/RConn1
  Battery_Cell22/RConn2 -- Conductive Heat Transfer18/LConn1 -- T19/RConn1
  Battery_Cell21/RConn1 -- Batt19/RConn1 -- Battery_Cell22/LConn1
  Battery_Cell14/LConn1 -- Batt22/RConn1 -- Battery_Cell24/RConn1
  Battery_Cell20/RConn2 -- Conductive Heat Transfer16/LConn1 -- T17/RConn1
  Battery_Cell13/RConn2 -- Conductive Heat Transfer12/LConn1 -- T13/RConn1
  Battery_Cell18/RConn2 -- Conductive Heat Transfer14/LConn1 -- T15/RConn1
  Battery_Cell16/RConn2 -- Conductive Heat Transfer23/LConn1 -- T24/RConn1
  Battery_Cell14/RConn2 -- Conductive Heat Transfer21/LConn1 -- T22/RConn1
  Battery_Cell20/RConn1 -- Batt18/RConn1 -- Battery_Cell21/LConn1
  Battery_Cell14/RConn1 -- Batt23/RConn1 -- Battery_Cell15/LConn1
  Battery_Cell19/RConn1 -- Batt17/RConn1 -- Battery_Cell20/LConn1
  Battery_Cell23/RConn2 -- Conductive Heat Transfer19/LConn1 -- T20/RConn1
  Battery_Cell24/RConn2 -- Conductive Heat Transfer20/LConn1 -- T21/RConn1
  Battery_Cell17/RConn2 -- Conductive Heat Transfer13/LConn1 -- T14/RConn1
  Battery_Cell15/RConn1 -- Batt24/RConn1 -- Battery_Cell16/LConn1
  Battery_Cell19/LConn1 -- Batt16/RConn1 -- Battery_Cell18/RConn1
  Battery_Cell19/RConn2 -- Conductive Heat Transfer15/LConn1 -- T16/RConn1
  Battery_Cell23/RConn1 -- Batt21/RConn1 -- Battery_Cell24/LConn1
  Battery_Cell21/RConn2 -- Conductive Heat Transfer17/LConn1 -- T18/RConn1
  Batt14/RConn1 -- Battery_Cell17/LConn1 -- Battery_Cell13/RConn1
  Batt20/RConn1 -- Battery_Cell23/LConn1 -- Battery_Cell22/RConn1
  Battery_Cell7/LConn2 -- s10/LConn1
  Battery_Cell9/LConn2 -- s6/LConn1
  Battery_Cell8/LConn2 -- s5/LConn1
  Battery_Cell12/LConn2 -- s9/LConn1
  Battery_Cell10/LConn2 -- s7/LConn1
  Batt13/RConn1 -- Battery_Cell13/LConn1 -- Battery_Cell12/RConn1
  Battery_Cell11/LConn2 -- s8/LConn1
  Battery_Cell9/RConn2 -- Conductive Heat Transfer8/LConn1 -- T9/RConn1
  Battery_Cell8/RConn2 -- Conductive Heat Transfer7/LConn1 -- T8/RConn1
  Battery_Cell11/RConn2 -- Conductive Heat Transfer10/LConn1 -- T11/RConn1
  Battery_Cell10/LConn1 -- Batt10/RConn1 -- Battery_Cell9/RConn1
  Battery_Cell10/RConn1 -- Batt11/RConn1 -- Battery_Cell11/LConn1
  Battery_Cell10/RConn2 -- Conductive Heat Transfer9/LConn1 -- T10/RConn1
  Battery_Cell8/RConn1 -- Batt9/RConn1 -- Battery_Cell9/LConn1
  Battery_Cell11/RConn1 -- Batt12/RConn1 -- Battery_Cell12/LConn1
  Battery_Cell12/RConn2 -- Conductive Heat Transfer11/LConn1 -- T12/RConn1
  Batt8/RConn1 -- Battery_Cell7/RConn1 -- Battery_Cell8/LConn1
  Battery_Cell7/RConn2 -- Conductive Heat Transfer6/LConn1 -- T7/RConn1
  Batt5/RConn1 -- Battery_Cell5/LConn1 -- Battery_Cell4/RConn1
  Batt6/RConn1 -- Battery_Cell6/LConn1 -- Battery_Cell5/RConn1
  Batt4/RConn1 -- Battery_Cell3/RConn1 -- Battery_Cell4/LConn1
  Battery_Cell1/RConn2 -- Conductive Heat Transfer/LConn1 -- T1/RConn1
  Battery_Cell5/RConn2 -- Conductive Heat Transfer4/LConn1 -- T5/RConn1
  Battery_Cell1/RConn1 -- Battery_Cell2/LConn1 -- Batt2/RConn1
  Battery_Cell6/RConn2 -- Conductive Heat Transfer5/LConn1 -- T6/RConn1
  Conductive Heat Transfer22/RConn1 -- Conductive Heat Transfer23/RConn1 -- Conductive Heat Transfer21/RConn1 -- Conductive Heat Transfer20/RConn1 -- Conductive Heat Transfer19/RConn1 -- Conductive Heat Transfer18/RConn1 -- Conductive Heat Transfer17/RConn1 -- Conductive Heat Transfer16/RConn1 -- Conductive Heat Transfer15/RConn1 -- Conductive Heat Transfer14/RConn1 -- Conductive Heat Transfer13/RConn1 -- Conductive Heat Transfer11/RConn1 -- Cold Plate/RConn1 -- Conductive Heat Transfer10/RConn1 -- Conductive Heat Transfer9/RConn1 -- Conductive Heat Transfer8/RConn1 -- Conductive Heat Transfer7/RConn1 -- Conductive Heat Transfer6/RConn1 -- Conductive Heat Transfer5/RConn1 -- Conductive Heat Transfer4/RConn1 -- Conductive Heat Transfer/RConn1 -- Conductive Heat Transfer1/RConn1 -- Conductive Heat Transfer2/RConn1 -- Conductive Heat Transfer3/RConn1 -- Conductive Heat Transfer12/RConn1
  Battery_Cell7/LConn1 -- Batt7/RConn1 -- Battery_Cell6/RConn1
  Batt1/RConn1 -- Battery_Cell1/LConn1
  Batt3/RConn1 -- Battery_Cell3/LConn1 -- Battery_Cell2/RConn1
  Battery_Cell1/LConn2 -- Subsystem/LConn1
  Battery_Cell2/LConn2 -- s/LConn1
  Battery_Cell3/LConn2 -- s1/LConn1
  Battery_Cell4/LConn2 -- s2/LConn1
  Battery_Cell5/LConn2 -- s3/LConn1
  Battery_Cell6/LConn2 -- s4/LConn1
  Battery_Cell3/RConn2 -- Conductive Heat Transfer2/LConn1 -- T3/RConn1
  Battery_Cell2/RConn2 -- Conductive Heat Transfer1/LConn1 -- T2/RConn1
  Battery_Cell4/RConn2 -- Conductive Heat Transfer3/LConn1 -- T4/RConn1
